simulink model "filter4_realization"  (R2020b)
settings: Solver=VariableStepAuto  StartTime=0.0  StopTime=10.0  RelTol=1e-3
settings Model: Creator=shivanshu shukla  LastModifiedBy=shivanshu shukla

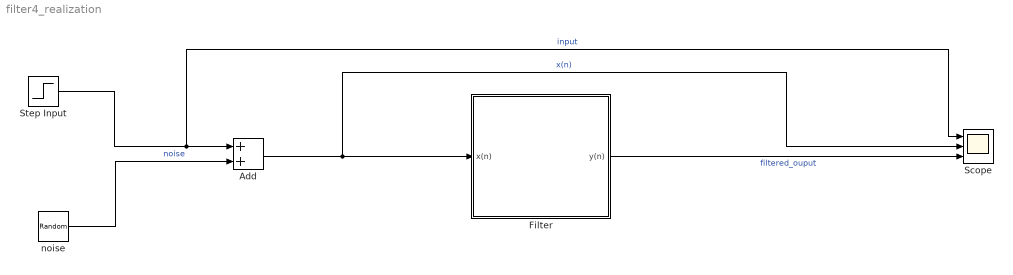
== system filter4_realization ==
  Add : Sum
  Filter : Subsystem
  Scope : Scope  NumInputPorts=3
  Step Input : Step  After=5  SampleTime=0
  noise : RandomNumber  SampleTime=0.1
  wires:
  Add/1 -> Scope/2, Filter/1(x(n))  "x(n)"
  Filter/1(y(n)) -> Scope/3  "filtered_ouput"
  noise/1 -> Add/2  "noise"
  Step Input/1 -> Scope/1, Add/1  "input"

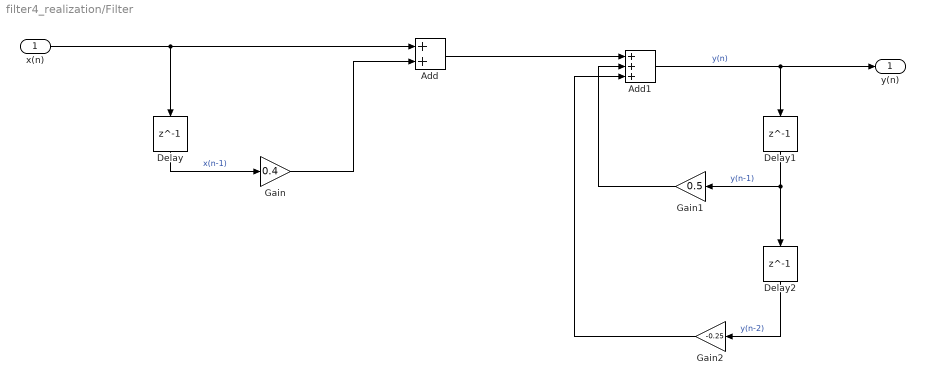
== system filter4_realization/Filter ==
  x(n) : Inport
  Add : Sum
  Add1 : Sum  Inputs=+++
  Delay : Delay  DelayLength=1
  Delay1 : Delay  DelayLength=1
  Delay2 : Delay  DelayLength=1
  Gain : Gain  Gain=0.4
  Gain1 : Gain  Gain=0.5
  Gain2 : Gain  Gain=-0.25
  y(n) : Outport
  wires:
  Add1/1 -> y(n)/1, Delay1/1  "y(n)"
  Gain1/1 -> Add1/2
  Add/1 -> Add1/1
  Delay2/1 -> Gain2/1  "y(n-2)"
  Gain2/1 -> Add1/3
  Gain/1 -> Add/2
  Delay1/1 -> Delay2/1, Gain1/1  "y(n-1)"
  x(n)/1 -> Add/1, Delay/1
  Delay/1 -> Gain/1  "x(n-1)"
